simulink model "lab1ex6"  (Simulink 6.0)
settings: Solver=ode45  StartTime=0.0  StopTime=10.0  RelTol=1e-3
settings Model: LastModifiedBy=student

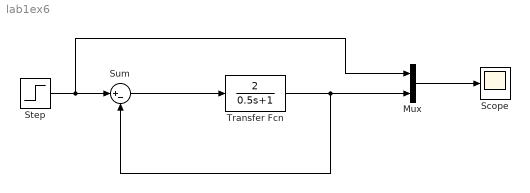
== system lab1ex6 ==
  Mux : Mux  Inputs=2
  Scope : Scope
  Step : Step  SampleTime=0
  Sum : Sum  Inputs=|+-
  Transfer Fcn : TransferFcn  Numerator=[2]  Denominator=[0.5 1]
  wires:
  Sum/1 -> Transfer Fcn/1
  Step/1 -> Sum/1, Mux/1
  Transfer Fcn/1 -> Mux/2, Sum/2
  Mux/1 -> Scope/1
